simulink model "IMUTest"  (R2021a)
settings: Solver=VariableStepAuto  StartTime=0.0  StopTime=10.0  RelTol=1e-3
libraries: simulink x7
settings Model: Creator=jmher  LastModifiedBy=jmher

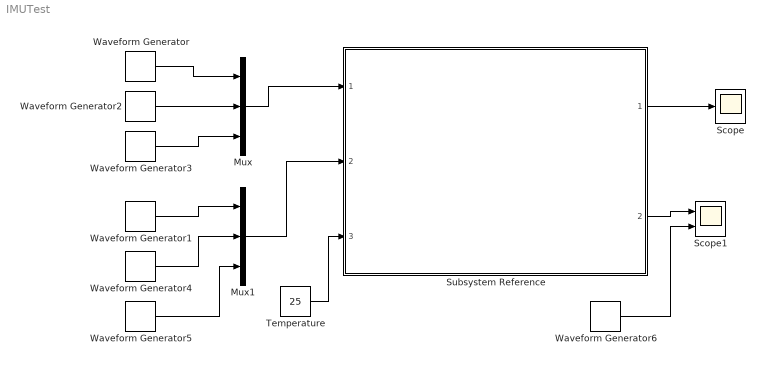
== system IMUTest ==
  Mux : Mux  Inputs=3
  Mux1 : Mux  Inputs=3
  Scope : Scope
  Scope1 : Scope  NumInputPorts=2
  Subsystem Reference : Subsystem  ReferencedSubsystem=IMU
  Temperature : Constant  Value=25
  Waveform Generator : simulink/Sources/Waveform Generator  OutMin=[]  OutMax=[]  OutDataTypeStr=double  SelectedSignal=1  Signals=sin(2,1,0)  BlockNames=MultiportSwitch_22b15b772c834b9  SampleTime=0.001
  Waveform Generator1 : simulink/Sources/Waveform Generator  OutMin=[]  OutMax=[]  OutDataTypeStr=double  SelectedSignal=1  Signals=sin(10,1,0)  BlockNames=MultiportSwitch_8d45418214b64e9  SampleTime=0.001
  Waveform Generator2 : simulink/Sources/Waveform Generator  OutMin=[]  OutMax=[]  OutDataTypeStr=double  SelectedSignal=1  Signals=sin(2,1,0)  BlockNames=MultiportSwitch_3c9d8708410d4c9  SampleTime=0.001
  Waveform Generator3 : simulink/Sources/Waveform Generator  OutMin=[]  OutMax=[]  OutDataTypeStr=double  SelectedSignal=1  Signals=sin(2,1,0)  BlockNames=MultiportSwitch_027c50d39e8e42e  SampleTime=0.001
  Waveform Generator4 : simulink/Sources/Waveform Generator  OutMin=[]  OutMax=[]  OutDataTypeStr=double  SelectedSignal=1  Signals=sin(10,1,0)  BlockNames=MultiportSwitch_22c75d545fcc434  SampleTime=0.001
  Waveform Generator5 : simulink/Sources/Waveform Generator  OutMin=[]  OutMax=[]  OutDataTypeStr=double  SelectedSignal=1  Signals=sin(10,1,0)  BlockNames=MultiportSwitch_0423a419685f425  SampleTime=0.001
  Waveform Generator6 : simulink/Sources/Waveform Generator  OutMin=[]  OutMax=[]  OutDataTypeStr=double  SelectedSignal=1  Signals=sin(10,1,0)  BlockNames=MultiportSwitch_0423a419685f425  SampleTime=1/40
  wires:
  Subsystem Reference/1 -> Scope/1
  Mux/1 -> Subsystem Reference/1
  Waveform Generator3/1 -> Mux/3
  Waveform Generator2/1 -> Mux/2
  Waveform Generator/1 -> Mux/1
  Mux1/1 -> Subsystem Reference/2
  Waveform Generator1/1 -> Mux1/1
  Waveform Generator4/1 -> Mux1/2
  Waveform Generator5/1 -> Mux1/3
  Subsystem Reference/2 -> Scope1/1
  Temperature/1 -> Subsystem Reference/3
  Waveform Generator6/1 -> Scope1/2
